simulink model "PWM"  (R2021a)
settings: Solver=VariableStepAuto  StartTime=0.0  StopTime=10.0  RelTol=1e-3
libraries: simulink x1
settings Model: Creator=ADMIN  LastModifiedBy=ADMIN

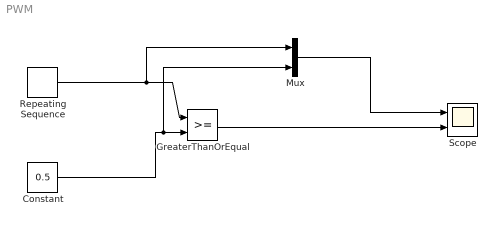
== system PWM ==
  Constant : Constant  Value=0.5
  GreaterThanOrEqual : RelationalOperator  OutDataTypeStr=boolean  RndMeth=Simplest
  Mux : Mux  Inputs=2
  Repeating Sequence : simulink/Sources/Repeating Sequence  rep_seq_t=[0 2]  rep_seq_y=[0 2]
  Scope : Scope  NumInputPorts=2
  wires:
  Repeating Sequence/1 -> Mux/1, GreaterThanOrEqual/1
  Constant/1 -> Mux/2, GreaterThanOrEqual/2
  GreaterThanOrEqual/1 -> Scope/2
  Mux/1 -> Scope/1
